simulink library "truck_lib"  (R2024a)
settings: Solver=VariableStepAuto  StartTime=0.0  StopTime=10.0  RelTol=1e-3
libraries: slpidlib x1
settings Model: Creator=adriaeik  LastModifiedBy=adriaeik

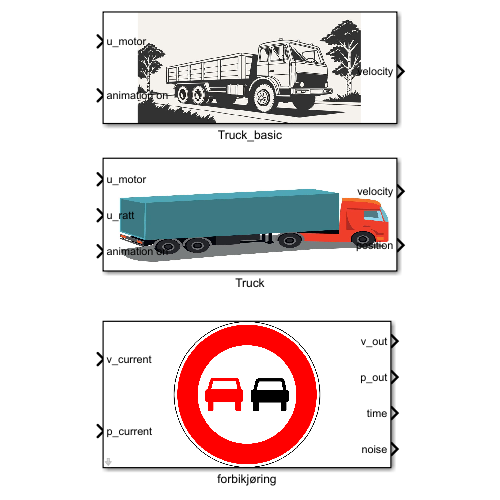
[thumbnail: Simulink's stored preview of the top-level diagram]
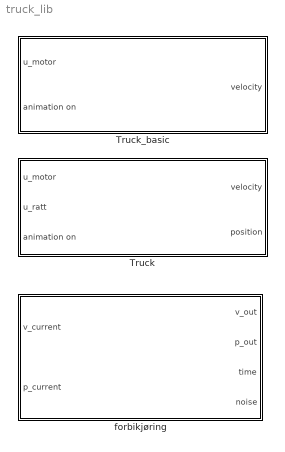
== system truck_lib ==
  Truck : Subsystem
      mask Display: image('truck_turn.png');
  Truck_basic : Subsystem
      mask Display: image('truck.png', [0,0,0,0,80,100]);
  forbikjøring : Subsystem  mask{speedlimit=15, wrooooom=25}
      mask Display: image('forbi.png', [0,0,0,0,80,100]);

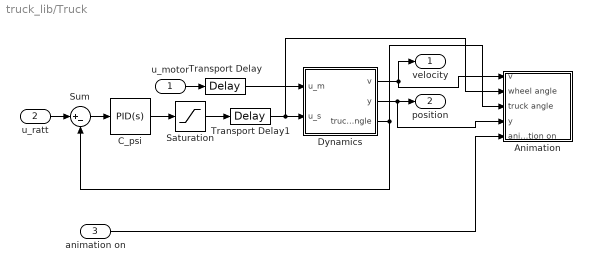
== system truck_lib/Truck ==
  u_motor : Inport
  u_ratt : Inport  Port=2
  animation on : Inport  Port=3
  Animation : Subsystem
  C_psi : slpidlib/PID Controller  Controller=PID  Form=Parallel  TimeDomain=Continuous-time  UseExternalTs=off  SampleTime=-1  IntegratorMethod=Forward Euler  FilterMethod=Forward Euler  ControllerParametersSource=internal  P=1  I=1  UseKiTs=off  D=0  UseExternalDerivativeSource=off  N=100  UseFilter=on  TunerSelectOption=Transfer Function Based (PID Tuner App)  InitialConditionSource=internal  InitialConditionForIntegrator=0  InitialConditionForFilter=0  DifferentiatorICPrevScaledInput=0  ExternalReset=none  TrackingMode=off  Kt=1  LimitOutput=off  SatLimitsSource=internal  UpperSaturationLimit=inf  LowerSaturationLimit=-inf  LinearizeAsGain=on  AntiWindupMode=none  Kb=1  LimitIntegrator=off  UpperIntegratorSaturationLimit=inf  LowerIntegratorSaturationLimit=-inf  POutMin=[]  POutMax=[]  IOutMin=[]  IOutMax=[]  DOutMin=[]  DOutMax=[]  NOutMin=[]  NOutMax=[]  SumOutMin=[]  SumOutMax=[]  SaturationOutMin=[]  SaturationOutMax=[]  PParamMin=[]  PParamMax=[]  IParamMin=[]  IParamMax=[]  DParamMin=[]  DParamMax=[]  NParamMin=[]  NParamMax=[]  KbParamMin=[]  KbParamMax=[]  KtParamMin=[]  KtParamMax=[]  KbOutMin=[]  KbOutMax=[]  KtOutMin=[]  KtOutMax=[]  IntegratorOutMin=[]  IntegratorOutMax=[]  FilterOutMin=[]  FilterOutMax=[]  SumI1OutMin=[]  SumI1OutMax=[]  SumI2OutMin=[]  SumI2OutMax=[]  SumI3OutMin=[]  SumI3OutMax=[]  SumI4OutMin=[]  SumI4OutMax=[]  SumDOutMin=[]  SumDOutMax=[]  DifferentiatorOutMin=[]  DifferentiatorOutMax=[]  FilterDiffOutCoefMin=[]  FilterDiffOutCoefMax=[]  ReciprocalOutMin=[]  ReciprocalOutMax=[]  SumDenOutMin=[]  SumDenOutMax=[]  SumNumOutMin=[]  SumNumOutMax=[]  DivideOutMin=[]  DivideOutMax=[]  UdiffTsProdOutMin=[]  UdiffTsProdOutMax=[]  NTsProdOutMin=[]  NTsProdOutMax=[]  UintegralTsProdOutMin=[]  UintegralTsProdOutMax=[]  UngainTsProdOutMin=[]  UngainTsProdOutMax=[]  ClampingZeroOutDataTypeStr=Inherit: Inherit via back propagation  ClampingZeroOutMin=[]  ClampingZeroOutMax=[]  FilterDenConstantOutDataTypeStr=Inherit: Inherit via back propagation  FilterDenConstantOutMin=[]  FilterDenConstantOutMax=[]  PCopyOutDataTypeStr=Inherit: Inherit via back propagation  PCopyOutMin=[]  PCopyOutMax=[]  NCopyOutDataTypeStr=Inherit: Inherit via back propagation  NCopyOutMin=[]  NCopyOutMax=[]  IntegratorContinuousStateAttributes=''  IntegratorStateMustResolveToSignalObject=off  IntegratorRTWStateStorageClass=Auto  FilterContinuousStateAttributes=''  FilterStateMustResolveToSignalObject=off  FilterRTWStateStorageClass=Auto  ParallelPVariant=InternalParameters  IdealPVariant=Disabled  IVariant=InternalParameters  DVariant=InternalParameters  IntegratorVariant=Continuous  SatVariant=Disabled  AWVariant=Passthrough  PCopyVariant=Disabled  TRVariant=Disabled  FdbkBlocksVariant=Forward  IdealPFdbkVariant=Disabled  SatFdbkVariant=Disabled  DerivativeFilterVariant=ContFilter  NVariant=InternalParameters  NCopyVariant=Disabled  FilterICVariant=InternalICsFilter  IntegratorICVariant=InternalICs  ExternalResetVariant=Disabled  TRSumVariant=Passthrough  SumFdbkVariant=Disabled  SumVariant=Sum_PID  TsampFilterVariant=InternalTs  TsampNgainVariant=Passthrough  TsampIntegralVariant=Disabled_SignalSpec  ExternalSaturationOutDataTypeStr=Inherit: Same as second input  DerivativeSourceVariant=ErrorSignal
  Dynamics : Subsystem  ClipboardFcn=parameters_truck.m
  Saturation : Saturate  UpperLimit=pi/4  LowerLimit=-pi/4
  Sum : Sum  Inputs=|+-
  Transport Delay : TransportDelay
  Transport Delay1 : TransportDelay  DelayTime=0.05
  velocity : Outport
  position : Outport  Port=2
  wires:
  Dynamics/2(y) -> position/1, Animation/4(y)
  u_ratt/1 -> Sum/1
  u_motor/1 -> Transport Delay/1
  Dynamics/3(truck angle) -> Sum/2, Animation/3(truck angle)
  Transport Delay1/1 -> Animation/2(wheel angle), Dynamics/2(u_s)
  Dynamics/1(v) -> velocity/1, Animation/1(v)
  C_psi/1 -> Saturation/1
  Sum/1 -> C_psi/1
  animation on/1 -> Animation/5(animation on)
  Transport Delay/1 -> Dynamics/1(u_m)
  Saturation/1 -> Transport Delay1/1

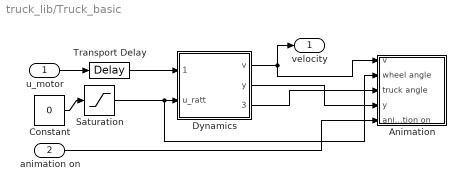
== system truck_lib/Truck_basic ==
  u_motor : Inport
  animation on : Inport  Port=2
  Animation : Subsystem
  Constant : Constant  Value=0
  Dynamics : Subsystem  ClipboardFcn=parameters_truck.m
  Saturation : Saturate  UpperLimit=pi/4  LowerLimit=-pi/4
  Transport Delay : TransportDelay
  velocity : Outport
  wires:
  Dynamics/2(y) -> Animation/4(y)
  Constant/1 -> Saturation/1
  u_motor/1 -> Transport Delay/1
  Dynamics/3(truck angle) -> Animation/3(truck angle)
  Saturation/1 -> Animation/2(wheel angle), Dynamics/2(u_ratt)
  Dynamics/1(v) -> velocity/1, Animation/1(v)
  animation on/1 -> Animation/5(animation on)
  Transport Delay/1 -> Dynamics/1(u_motor)

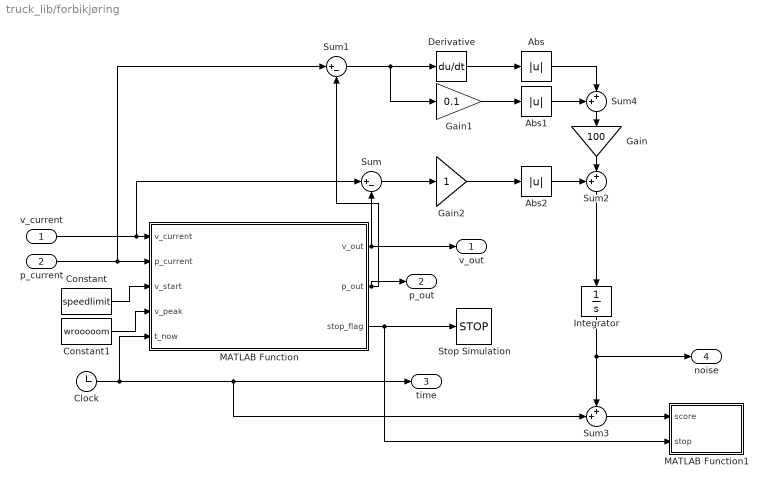
== system truck_lib/forbikjøring ==
  v_current : Inport
  p_current : Inport  Port=2
  Abs : Abs  SaturateOnIntegerOverflow=off
  Abs1 : Abs  SaturateOnIntegerOverflow=off
  Abs2 : Abs  SaturateOnIntegerOverflow=off
  Clock : Clock
  Constant : Constant  Value=speedlimit
  Constant1 : Constant  Value=wrooooom
  Derivative : Derivative
  Gain : Gain  Gain=100
  Gain1 : Gain  Gain=0.1
  Gain2 : Gain
  Integrator : Integrator
  MATLAB Function : MATLAB Function  TreatAsAtomicUnit=on
  MATLAB Function1 : MATLAB Function  TreatAsAtomicUnit=on
  Stop Simulation : Stop
  Sum : Sum  Inputs=|+-
  Sum1 : Sum  Inputs=|+-
  Sum2 : Sum  Inputs=++|
  Sum3 : Sum  Inputs=++|
  Sum4 : Sum  Inputs=++|
  v_out : Outport
  p_out : Outport  Port=2
  time : Outport  Port=3
  noise : Outport  Port=4
  wires:
  MATLAB Function/3(stop_flag) -> Stop Simulation/1, MATLAB Function1/2(stop)
  v_current/1 -> MATLAB Function/1(v_current), Sum/1
  MATLAB Function/1(v_out) -> Sum/2, v_out/1
  Clock/1 -> MATLAB Function/5(t_now), Sum3/2, time/1
  Constant/1 -> MATLAB Function/3(v_start)
  Constant1/1 -> MATLAB Function/4(v_peak)
  Sum1/1 -> Gain1/1, Derivative/1
  p_current/1 -> Sum1/1, MATLAB Function/2(p_current)
  MATLAB Function/2(p_out) -> Sum1/2, p_out/1
  Sum3/1 -> MATLAB Function1/1(score)
  Gain/1 -> Sum2/2
  Integrator/1 -> noise/1, Sum3/1
  Sum/1 -> Gain2/1
  Sum4/1 -> Gain/1
  Abs/1 -> Sum4/2
  Derivative/1 -> Abs/1
  Gain1/1 -> Abs1/1
  Abs1/1 -> Sum4/1
  Sum2/1 -> Integrator/1
  Gain2/1 -> Abs2/1
  Abs2/1 -> Sum2/1

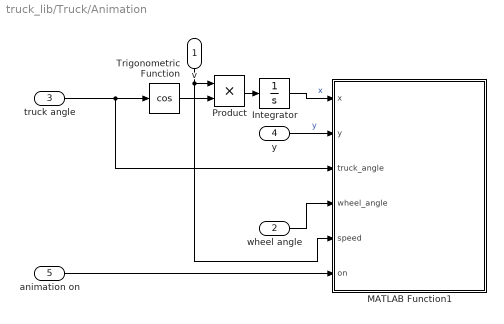
== system truck_lib/Truck/Animation ==
  v : Inport
  wheel angle : Inport  Port=2
  truck angle : Inport  Port=3
  y : Inport  Port=4
  animation on : Inport  Port=5
  Integrator : Integrator
  MATLAB Function1 : MATLAB Function  TreatAsAtomicUnit=on  SystemSampleTime=1/30
  Product : Product
  Trigonometric Function : Trigonometry  Operator=cos
  wires:
  Product/1 -> Integrator/1
  Trigonometric Function/1 -> Product/2
  v/1 -> MATLAB Function1/5(speed), Product/1
  y/1 -> MATLAB Function1/2(y)  "y"
  Integrator/1 -> MATLAB Function1/1(x)  "x"
  truck angle/1 -> MATLAB Function1/3(truck_angle), Trigonometric Function/1
  wheel angle/1 -> MATLAB Function1/4(wheel_angle)
  animation on/1 -> MATLAB Function1/6(on)

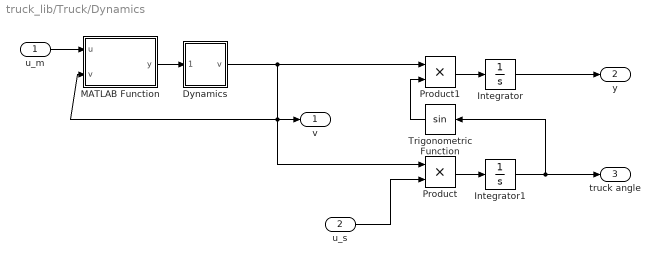
== system truck_lib/Truck/Dynamics ==
  u_m : Inport
  u_s : Inport  Port=2
  Dynamics : Subsystem  ClipboardFcn=parameters_truck.m
  Integrator : Integrator  InitialCondition=-2
  Integrator1 : Integrator
  MATLAB Function : MATLAB Function  TreatAsAtomicUnit=on
  Product : Product
  Product1 : Product
  Trigonometric Function : Trigonometry
  v : Outport
  y : Outport  Port=2
  truck angle : Outport  Port=3
  wires:
  Integrator/1 -> y/1
  Product/1 -> Integrator1/1
  Product1/1 -> Integrator/1
  Trigonometric Function/1 -> Product1/2
  u_s/1 -> Product/2
  Integrator1/1 -> truck angle/1, Trigonometric Function/1
  MATLAB Function/1(y) -> Dynamics/1(u_m)
  u_m/1 -> MATLAB Function/1(u)
  Dynamics/1(v) -> Product1/1, Product/1, MATLAB Function/2(v), v/1

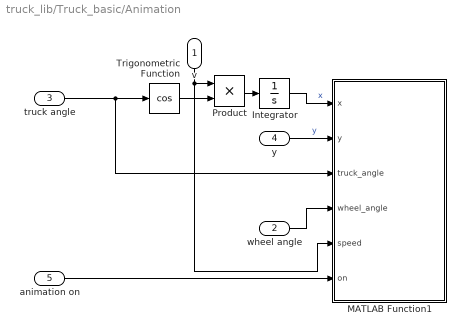
== system truck_lib/Truck_basic/Animation ==
  v : Inport
  wheel angle : Inport  Port=2
  truck angle : Inport  Port=3
  y : Inport  Port=4
  animation on : Inport  Port=5
  Integrator : Integrator
  MATLAB Function1 : MATLAB Function  TreatAsAtomicUnit=on  SystemSampleTime=1/30
  Product : Product
  Trigonometric Function : Trigonometry  Operator=cos
  wires:
  Product/1 -> Integrator/1
  Trigonometric Function/1 -> Product/2
  v/1 -> MATLAB Function1/5(speed), Product/1
  y/1 -> MATLAB Function1/2(y)  "y"
  Integrator/1 -> MATLAB Function1/1(x)  "x"
  truck angle/1 -> MATLAB Function1/3(truck_angle), Trigonometric Function/1
  wheel angle/1 -> MATLAB Function1/4(wheel_angle)
  animation on/1 -> MATLAB Function1/6(on)

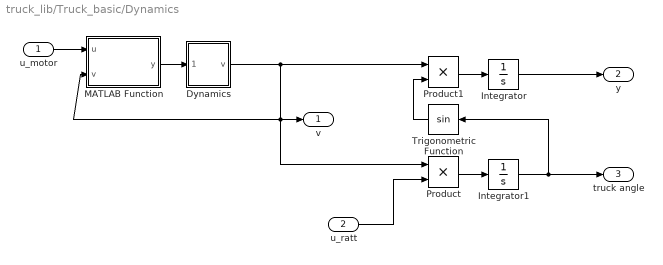
== system truck_lib/Truck_basic/Dynamics ==
  u_motor : Inport
  u_ratt : Inport  Port=2
  Dynamics : Subsystem  ClipboardFcn=parameters_truck.m
  Integrator : Integrator  InitialCondition=-2
  Integrator1 : Integrator
  MATLAB Function : MATLAB Function  TreatAsAtomicUnit=on
  Product : Product
  Product1 : Product
  Trigonometric Function : Trigonometry
  v : Outport
  y : Outport  Port=2
  truck angle : Outport  Port=3
  wires:
  Integrator/1 -> y/1
  Product/1 -> Integrator1/1
  Product1/1 -> Integrator/1
  Trigonometric Function/1 -> Product1/2
  u_ratt/1 -> Product/2
  Integrator1/1 -> truck angle/1, Trigonometric Function/1
  MATLAB Function/1(y) -> Dynamics/1(u_m)
  u_motor/1 -> MATLAB Function/1(u)
  Dynamics/1(v) -> Product1/1, Product/1, MATLAB Function/2(v), v/1

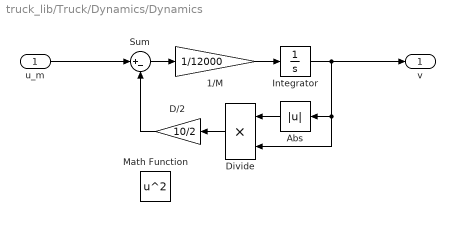
== system truck_lib/Truck/Dynamics/Dynamics ==
  u_m : Inport
  1/M : Gain  Gain=1/12000
  Abs : Abs  SaturateOnIntegerOverflow=off
  D/2 : Gain  Gain=10/2
  Divide : Product  Inputs=**
  Integrator : Integrator
  Math Function : Math  Operator=square  SignedPower=on
  Sum : Sum  Inputs=|+-
  v : Outport
  wires:
  Integrator/1 -> v/1, Abs/1, Divide/2
  Sum/1 -> 1/M/1
  u_m/1 -> Sum/1
  1/M/1 -> Integrator/1
  Divide/1 -> D/2/1
  D/2/1 -> Sum/2
  Abs/1 -> Divide/1

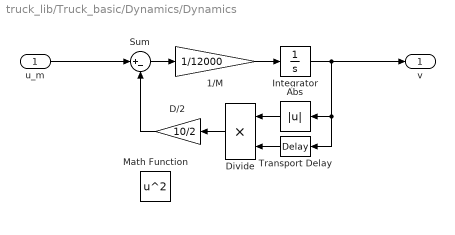
== system truck_lib/Truck_basic/Dynamics/Dynamics ==
  u_m : Inport
  1/M : Gain  Gain=1/12000
  Abs : Abs  SaturateOnIntegerOverflow=off
  D/2 : Gain  Gain=10/2
  Divide : Product  Inputs=**
  Integrator : Integrator
  Math Function : Math  Operator=square  SignedPower=on
  Sum : Sum  Inputs=|+-
  Transport Delay : TransportDelay
  v : Outport
  wires:
  Integrator/1 -> v/1, Transport Delay/1, Abs/1
  Sum/1 -> 1/M/1
  u_m/1 -> Sum/1
  1/M/1 -> Integrator/1
  Divide/1 -> D/2/1
  D/2/1 -> Sum/2
  Abs/1 -> Divide/1
  Transport Delay/1 -> Divide/2

== matlab function truck_lib/Truck_basic/Dynamics/MATLAB Function ==
  data: u input; y output; v input
function y = saturation(u,v)
    Pmax = 400000;
    epsilon = 0.1;
    
    sat = Pmax/sqrt(v^2+epsilon);
    y = max(min(u,sat),-sat);

== matlab function truck_lib/Truck/Animation/MATLAB Function1 ==
  settings: updateMethod=DISCRETE
  data: x input; y input; truck_angle input; wheel_angle input; speed input; on input
function plot_truck(x, y, truck_angle, wheel_angle, speed, on)
    
        coder.extrinsic('figure', 'clf', 'grid', 'hold', 'daspect', 'xlim', 'ylim', ...
                        'plot', 'rectangle', 'hgtransform', 'makehgtform', ...
                        'set', 'get', 'gca', 'text', 'ishandle', ...
                        'sprintf', 'rad2deg');
    if on
        l = 8;
    
        % Initier eller hent eksisterande figur
        fig = findobj('Type', 'figure', 'Name', 'TruckPlot');
        if isempty(fig)
            fig = figure('Name', 'TruckPlot', 'Position', [100, 100, 1500, 500]);
        else
            figure(fig);
        end
        clf; grid on; hold on; daspect([1, 1, 1]);
        xlim([-20, 50] + x)
        ylim([-10, 10] + y)
    
        % Veg
        plot([-5000, 5000], [-4, -4], 'k', 'linewidth', 3);
        plot([-5000, 5000], [4, 4], 'k', 'linewidth', 3);
        plot([-5000, 5000], [0, 0], 'y', 'linewidth', 3);
    
        % Truck
        Truck = hgtransform('Parent', gca);
        Left_front_wheel = hgtransform('Parent', Truck);
        Right_front_wheel = hgtransform('Parent', Truck);
    
        % Hjul bak
        rectangle('Position', [l/6, -l/100, l/8, l/40], 'Parent', Truck, 'EdgeColor', 'k', 'LineWidth', 2, 'FaceColor', 'w');
        rectangle('Position', [l/6, l - 2*l/3 - (l/40 - l/100), l/8, l/40], 'Parent', Truck, 'EdgeColor', 'k', 'LineWidth', 2, 'FaceColor', 'w');
    
        % Hjul fram
        rectangle('Position', [2*l/3 + l/20, -l/100, l/8, l/40], 'Parent', Right_front_wheel, 'EdgeColor', 'k', 'LineWidth', 2, 'FaceColor', 'w');
        rectangle('Position', [2*l/3 + l/20, l - 2*l/3 - (l/40 - l/100), l/8, l/40], 'Parent', Left_front_wheel, 'EdgeColor', 'k', 'LineWidth', 2, 'FaceColor', 'w');
    
        % Kropp
        rectangle('Position', [0, 0, 11*l/18, l - 2*l/3], 'Parent', Truck, 'EdgeColor', 'k', 'LineWidth', 2, 'FaceColor', 'w');
        rectangle('Position', [2*l/3, 0, l - 2*l/3, l - 2*l/3], 'Parent', Truck, 'EdgeColor', 'k', 'LineWidth', 2, 'FaceColor', 'w');
        rectangle('Position', [11*l/18, 3*l/8 - l/3, 2*l/3 - 11*l/18, l - 3*l/4], 'Parent', Truck, 'EdgeColor', 'k', 'LineWidth', 2, 'FaceColor', 'w');
        rectangle('Position', [7*l/8, 0, l/8, l - 2*l/3], 'Parent', Truck, 'EdgeColor', 'k', 'LineWidth', 2, 'FaceColor', 'w');
    
        % Fartstekst
        text(l/9, 2*l/7, 0, sprintf('%.2f m/s', speed), ...
             'Parent', Truck, ...
             'FontSize', 12, ...
             'FontWeight', 'bold', ...
             'Rotation', rad2deg(truck_angle));
    
        % Posisjon og rotasjon
        set(Truck, 'Matrix', makehgtform( ...
            'translate', [x, y, 0], ...
            'zrotate', truck_angle, ...
            'translate', [-l/6 - l/16, -l/2 + l/3, 0]));
    
        % Hjulrotasjon
        set(Left_front_wheel, 'Matrix', makehgtform( ...
            'translate', -[-(2*l/3 + l/20) - l/16, l/100 - l/80, 0], ...
            'zrotate', -wheel_angle, ...
            'translate', [-(2*l/3 + l/20) - l/16, l/100 - l/80, 0]));
    
        set(Right_front_wheel, 'Matrix', makehgtform( ...
            'translate', -[-(2*l/3 + l/20) - l/16, -(l - 2*l/3 - (l/40 - l/100)) - l/80, 0], ...
            'zrotate', -wheel_angle, ...
            'translate', [-(2*l/3 + l/20) - l/16, -(l - 2*l/3 - (l/40 - l/100)) - l/80, 0]));
    
        drawnow;
    end
end

== matlab function truck_lib/Truck_basic/Animation/MATLAB Function1 ==
  settings: updateMethod=DISCRETE
  data: x input; y input; truck_angle input; wheel_angle input; speed input; on input
function plot_truck(x, y, truck_angle, wheel_angle, speed, on)
    
        coder.extrinsic('figure', 'clf', 'grid', 'hold', 'daspect', 'xlim', 'ylim', ...
                        'plot', 'rectangle', 'hgtransform', 'makehgtform', ...
                        'set', 'get', 'gca', 'text', 'ishandle', ...
                        'sprintf', 'rad2deg');
    if on
        l = 8;
    
        % Initier eller hent eksisterande figur
        fig = findobj('Type', 'figure', 'Name', 'TruckPlot');
        if isempty(fig)
            fig = figure('Name', 'TruckPlot', 'Position', [100, 100, 1500, 500]);
        else
            figure(fig);
        end
        clf; grid on; hold on; daspect([1, 1, 1]);
        xlim([-20, 50] + x)
        ylim([-10, 10] + y)
    
        % Veg
        plot([-5000, 5000], [-4, -4], 'k', 'linewidth', 3);
        plot([-5000, 5000], [4, 4], 'k', 'linewidth', 3);
        plot([-5000, 5000], [0, 0], 'y', 'linewidth', 3);
    
        % Truck
        Truck = hgtransform('Parent', gca);
        Left_front_wheel = hgtransform('Parent', Truck);
        Right_front_wheel = hgtransform('Parent', Truck);
    
        % Hjul bak
        rectangle('Position', [l/6, -l/100, l/8, l/40], 'Parent', Truck, 'EdgeColor', 'k', 'LineWidth', 2, 'FaceColor', 'w');
        rectangle('Position', [l/6, l - 2*l/3 - (l/40 - l/100), l/8, l/40], 'Parent', Truck, 'EdgeColor', 'k', 'LineWidth', 2, 'FaceColor', 'w');
    
        % Hjul fram
        rectangle('Position', [2*l/3 + l/20, -l/100, l/8, l/40], 'Parent', Right_front_wheel, 'EdgeColor', 'k', 'LineWidth', 2, 'FaceColor', 'w');
        rectangle('Position', [2*l/3 + l/20, l - 2*l/3 - (l/40 - l/100), l/8, l/40], 'Parent', Left_front_wheel, 'EdgeColor', 'k', 'LineWidth', 2, 'FaceColor', 'w');
    
        % Kropp
        rectangle('Position', [0, 0, 11*l/18, l - 2*l/3], 'Parent', Truck, 'EdgeColor', 'k', 'LineWidth', 2, 'FaceColor', 'w');
        rectangle('Position', [2*l/3, 0, l - 2*l/3, l - 2*l/3], 'Parent', Truck, 'EdgeColor', 'k', 'LineWidth', 2, 'FaceColor', 'w');
        rectangle('Position', [11*l/18, 3*l/8 - l/3, 2*l/3 - 11*l/18, l - 3*l/4], 'Parent', Truck, 'EdgeColor', 'k', 'LineWidth', 2, 'FaceColor', 'w');
        rectangle('Position', [7*l/8, 0, l/8, l - 2*l/3], 'Parent', Truck, 'EdgeColor', 'k', 'LineWidth', 2, 'FaceColor', 'w');
    
        % Fartstekst
        text(l/9, 2*l/7, 0, sprintf('%.2f m/s', speed), ...
             'Parent', Truck, ...
             'FontSize', 12, ...
             'FontWeight', 'bold', ...
             'Rotation', rad2deg(truck_angle));
    
        % Posisjon og rotasjon
        set(Truck, 'Matrix', makehgtform( ...
            'translate', [x, y, 0], ...
            'zrotate', truck_angle, ...
            'translate', [-l/6 - l/16, -l/2 + l/3, 0]));
    
        % Hjulrotasjon
        set(Left_front_wheel, 'Matrix', makehgtform( ...
            'translate', -[-(2*l/3 + l/20) - l/16, l/100 - l/80, 0], ...
            'zrotate', -wheel_angle, ...
            'translate', [-(2*l/3 + l/20) - l/16, l/100 - l/80, 0]));
    
        set(Right_front_wheel, 'Matrix', makehgtform( ...
            'translate', -[-(2*l/3 + l/20) - l/16, -(l - 2*l/3 - (l/40 - l/100)) - l/80, 0], ...
            'zrotate', -wheel_angle, ...
            'translate', [-(2*l/3 + l/20) - l/16, -(l - 2*l/3 - (l/40 - l/100)) - l/80, 0]));
    
        drawnow;
    end
end

== matlab function truck_lib/Truck/Dynamics/MATLAB Function ==
  data: u input; y output; v input
function y = saturation(u,v)
    Pmax = 400000;
    epsilon = 0.1;
    
    sat = Pmax/sqrt(v^2+epsilon);
    y = max(min(u,sat),-sat);

== matlab function truck_lib/forbikjøring/MATLAB Function ==
  settings: updateMethod=DISCRETE
  data: v_current input; p_current input; v_out output; p_out output; stop_flag output; v_start input; v_peak input; t_now input
function [v_out, p_out, stop_flag] = forbikjoring_controller(v_current, p_current, v_start, v_peak, t_now)
%#codegen
tol = 0.04;
delay = 1.0;
persistent state t_reached
if isempty(state)
    state = 0;
    t_reached = 0;
end

% Standard output
v_out = v_start;
p_out = -2;
stop_flag = 0;

switch state
    case 0  % Startfase: vent på å nå v_start
        v_out = v_start;
        p_out = -2;
        if v_current >= v_start
            state = 1;
        end

    case 1  % Sving ut
        v_out = v_peak;
        p_out = 2;
        if abs(v_current - v_out) < tol && abs(abs(p_current) - abs(p_out)) < tol
            state = 2;
        end

    case 2  % Sving tilbake
        v_out = v_start;
        p_out = -2;
        if abs(v_current - v_out) < tol && abs(abs(p_current) - abs(p_out)) < tol
            t_reached = t_now; % Start forsinkelsestid
            state = 3;
        end

    case 3  % Vent 1 sekund før stopp
        v_out = v_start;
        p_out = -2;
        if (t_now - t_reached) >= delay
            stop_flag = 1;
        end
end

== matlab function truck_lib/forbikjøring/MATLAB Function1 ==
  data: score input; stop input
function fcn(score, stop)
if score == inf || ~stop
    score = 9999999;
end
 assignin('base', 'score', score);
